simulink model "vechicle_detector_using_simulink"  (R2023a)
settings: Solver=FixedStepAuto  StartTime=0.0  StopTime=inf  RelTol=1e-3
libraries: dspvision x1, visionanalysis x1
settings Model: Creator=The MathWorks, Inc.
settings SolverCC: AlgebraicLoopSolver=TrustRegion
settings OptimizationCC: ReuseModelBlockBuffer=off  ZeroExternalMemoryAtStartup=off  ZeroInternalMemoryAtStartup=off  InitFltsAndDblsToZero=on
settings DebuggingCC: UnconnectedInputMsg=warning  UnconnectedOutputMsg=warning  UnconnectedLineMsg=warning  SymbolicDimsDataTypeCodeGenerationDiagnostic=none  IntegerSaturationMsg=none
settings HardwareCC: ProdLongLongMode=on  TargetLongLongMode=on
settings ModelReferenceCC: EnableRefExpFcnMdlSchedulingChecks=on  ModelReferencePassRootInputsByReference=off
settings RTWCC: TargetLang=C++  DLTargetLibrary=mkl-dnn  DLArmComputeVersion=19.05
settings GRTTargetCC: TargetLangStandard=C++11 (ISO)  MatFileLogging=off  CodeInterfacePackaging=C++ class

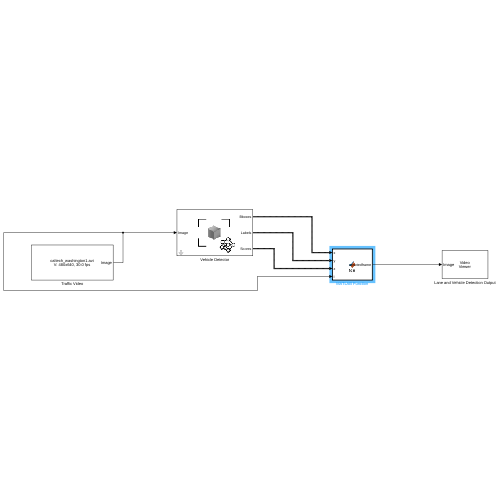
[thumbnail: Simulink's stored preview of the top-level diagram]
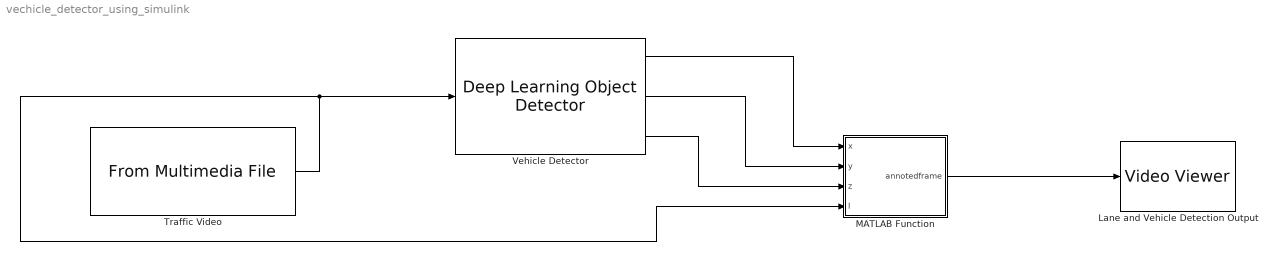
== system vechicle_detector_using_simulink ==
  Lane and Vehicle Detection Output : VideoViewer  FigPos=[505 794 664 500]
  MATLAB Function : MATLAB Function  TreatAsAtomicUnit=on
  Traffic Video : dspvision/From Multimedia File  inputFilename=caltech_washington1.avi  readRange=[1 Inf]  loop=on  numPlays=inf  outputStreams=Video only  videoDataType=single  audioDataType=int16  inheritSampleTime=on  userDefinedSampleTime=1/30  noAudioOutput=off  isIntensityVideo=off  fourcc=RGB  colorVideoFormat=One multidimensional signal  outputEOF=off  dataOrg=Column-major  audioFrameSize=1024  computeAudioFrameSize=off  outSamplingMode=Sample based
  Vehicle Detector : visionanalysis/Deep Learning Object Detector  Detector=Detector from MAT-file  DetectorFunction=untitled  DetectorFilePath=/MATLAB Drive/Examples/R2023a/deeplearning_shared/ObjectDetectionUsingYOLOV3DeepLearningExample/yolov3SqueezeNetVehicleExample_21aSPKG.mat  MaxDetections=20  Bboxes=on  Scores=on  UseROI=off  ROI=[1 1 100 100]  Threshold=0.3  NumStrongestRegions=2000  UseMinSize=off  MinSize=[1 1]  UseMaxSize=off  MaxSize=[50 50]  ForceInterpretedSim=off
  wires:
  Traffic Video/1 -> MATLAB Function/4(I), Vehicle Detector/1
  Vehicle Detector/1 -> MATLAB Function/1(x)
  Vehicle Detector/2 -> MATLAB Function/2(y)
  Vehicle Detector/3 -> MATLAB Function/3(z)
  MATLAB Function/1(annotedframe) -> Lane and Vehicle Detection Output/1

== matlab function vechicle_detector_using_simulink/MATLAB Function ==
  data: x input; annotedframe output; y input; z input; I input
function annotedframe = fcn(x,y,z,I)

bboxes=x;
scores=z;
labels=y;
annotedframe=insertObjectAnnotation(I,"rectangle",bboxes,scores);


end
